simulink model "ssc_helmet_uv_chamber"  (R2019b)
settings: Solver=VariableStepAuto  StartTime=0.0  StopTime=30  RelTol=1e-3  AbsTol=1e-3
undefined symbols (not defined in the file): sigbuilder_block
libraries: fl_lib x8, nesl_utility x7
(part 2 of 2)

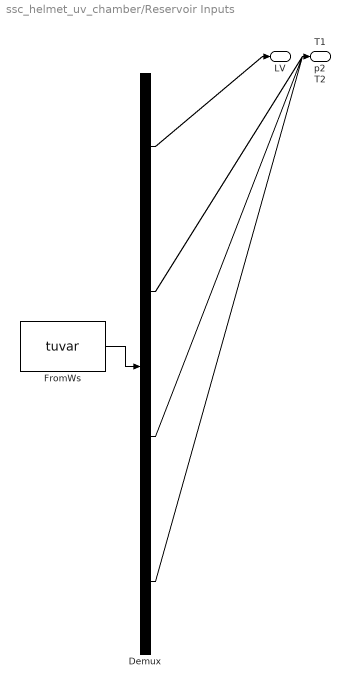
== system ssc_helmet_uv_chamber/Reservoir Inputs ==
  Demux : Demux  Tag=STV Demux
  FromWs : FromWorkspace  Tag=STV FromWs  VariableName=tuvar  SampleTime=0
      SigBuilderData=|
      | common.afterFinalStr = 'Extrapolate'
      | common.sampleTime = 0
      | dataSet.timeRange = [0 30]
      | dataSet.name = 'Imported_Group 1'
      | sbobj.Groups.Name = 'Imported_Group 1'
      | sbobj.Groups.Signals(1).Name = 'LV'
      | sbobj.Groups.Signals(1).XData = [0 3.92131600466e-08 1.1763948014e-07 2.89115827095e-07 4.75637635852e-07 6.62159444609e-07 1.07170365719e-06 1.48124786977e-06 1.89079208235e-06 2.30033629493e-06 3.42013773531e-06 4.53993917569e-06 ... (1888 elements, 1x1888)]
      | sbobj.Groups.Signals(1).YData = [0.002001 0.002001 0.002001 0.002001 0.002001 0.002001 0.00200100000001 0.00200100000002 0.00200100000004 0.00200100000005 0.00200100000012 0.00200100000021 ... (1888 elements, 1x1888)]
      | sbobj.Groups.Signals(2).Name = 'p2'
      | sbobj.Groups.Signals(2).XData = [0 30]
      | sbobj.Groups.Signals(2).YData = [0.101325 0.101325]
      | sbobj.Groups.Signals(3).Name = 'T1'
      | sbobj.Groups.Signals(3).XData = [0 30]
      | sbobj.Groups.Signals(3).YData = [310 310]
      | sbobj.Groups.Signals(4).Name = 'T2'
      | sbobj.Groups.Signals(4).XData = [0 30]
      | sbobj.Groups.Signals(4).YData = [300 300]
      | sbobj.Groups.TimeRange = [0 30]
  LV : Outport  Tag=STV Outport  VectorParamsAs1DForOutWhenUnconnected=off
  p2 : Outport  Tag=STV Outport  Port=2
  T1 : Outport  Tag=STV Outport  Port=3
  T2 : Outport  Tag=STV Outport  Port=4
  wires:
  FromWs/1 -> Demux/1
  Demux/1 -> LV/1
  Demux/2 -> p2/1
  Demux/3 -> T1/1
  Demux/4 -> T2/1

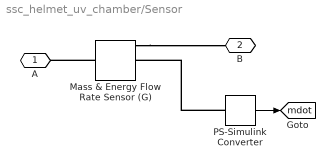
== system ssc_helmet_uv_chamber/Sensor ==
  Mass & Energy Flow Rate Sensor (G) : fl_lib/Gas/Sensors/Mass & Energy Flow Rate Sensor (G)
      settings: SourceProductName=Simscape  SourceProductBaseCode=SS  InternalSimscapePortConfiguration="{\"Bottom\":[],\"Left\":[{\"id\":\"A\",\"label\":\"A\",\"type\":\"foundation.gas.gas\"}],\"Right\":[{\"id\":\"B\",\"label\":\"B\",\"type\":\"foundation.gas.gas\"},{\"id\":\"M\",\"label\":\"M\",\"type\":\"output\"},{\"id\":\"PHI\",\"label\":\"Phi\",\"type\":\"output\"}],\"Top\":[]}"
  PS-Simulink Converter : nesl_utility/PS-Simulink Converter  PhysicalDomain=network_engine_domain  SubClassName=ps_output  LeftPortType=input  RightPortType=output  PseudoPeriodic=off  Frequencies=[]  Unit=kg/s  AffineConversion=off
  A : PMIOPort  Side=Left
  B : PMIOPort  Port=2  Side=Right
  tag scope: mdot=global
  wires:
  PS-Simulink Converter/1 -> [mdot]
  connections:
  PS-Simulink Converter/LConn1 -- Mass & Energy Flow Rate Sensor (G)/RConn2
  Mass & Energy Flow Rate Sensor (G)/LConn1 -- A/RConn1
  Mass & Energy Flow Rate Sensor (G)/RConn1 -- B/RConn1

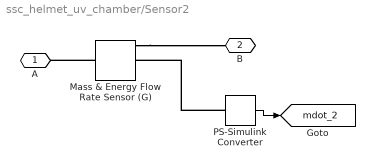
== system ssc_helmet_uv_chamber/Sensor2 ==
  Mass & Energy Flow Rate Sensor (G) : fl_lib/Gas/Sensors/Mass & Energy Flow Rate Sensor (G)
      settings: SourceProductName=Simscape  SourceProductBaseCode=SS  InternalSimscapePortConfiguration="{\"Bottom\":[],\"Left\":[{\"id\":\"A\",\"label\":\"A\",\"type\":\"foundation.gas.gas\"}],\"Right\":[{\"id\":\"B\",\"label\":\"B\",\"type\":\"foundation.gas.gas\"},{\"id\":\"M\",\"label\":\"M\",\"type\":\"output\"},{\"id\":\"PHI\",\"label\":\"Phi\",\"type\":\"output\"}],\"Top\":[]}"
  PS-Simulink Converter : nesl_utility/PS-Simulink Converter  PhysicalDomain=network_engine_domain  SubClassName=ps_output  LeftPortType=input  RightPortType=output  PseudoPeriodic=off  Frequencies=[]  Unit=kg/s  AffineConversion=off
  A : PMIOPort  Side=Left
  B : PMIOPort  Port=2  Side=Right
  tag scope: mdot_2=global
  wires:
  PS-Simulink Converter/1 -> [mdot_2]
  connections:
  PS-Simulink Converter/LConn1 -- Mass & Energy Flow Rate Sensor (G)/RConn2
  Mass & Energy Flow Rate Sensor (G)/LConn1 -- A/RConn1
  Mass & Energy Flow Rate Sensor (G)/RConn1 -- B/RConn1
